simulink model "Driver_Fault_triggers"  (R2016a)
settings: Solver=VariableStepAuto  StartTime=0.0  StopTime=10.0  RelTol=1e-3
libraries: simulink x6
settings Model: Creator=ullek  LastModifiedBy=ullek

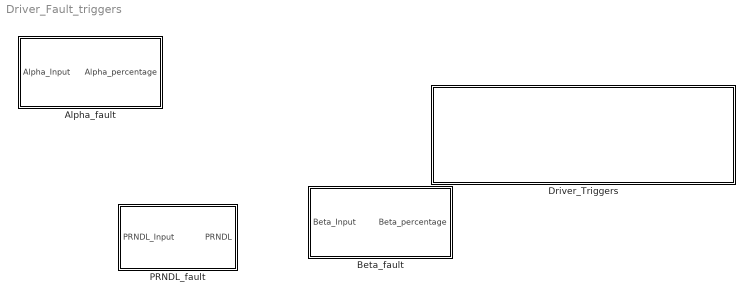
== system Driver_Fault_triggers ==
  Alpha_fault : Subsystem
  Beta_fault : Subsystem
  Driver_Triggers : Subsystem
  PRNDL_fault : Subsystem
  wires:
  ? -> Alpha_fault/1(Alpha_Input)  "Alpha_percentage"

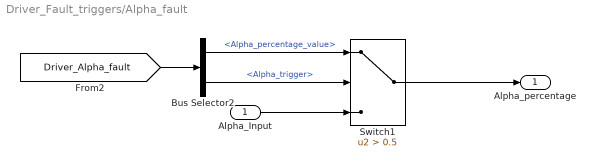
== system Driver_Fault_triggers/Alpha_fault ==
  Alpha_Input : Inport
  Bus Selector2 : BusSelector  OutputSignals=Alpha_percentage_value,Alpha_trigger
  Switch1 : Switch  Criteria=u2 > Threshold  Threshold=0.5
  Alpha_percentage : Outport
  wires:
  Alpha_Input/1 -> Switch1/3
  Switch1/1 -> Alpha_percentage/1
  Bus Selector2/2 -> Switch1/2  "<Alpha_trigger>"
  [Driver_Alpha_fault] -> Bus Selector2/1
  Bus Selector2/1 -> Switch1/1  "<Alpha_percentage_value>"

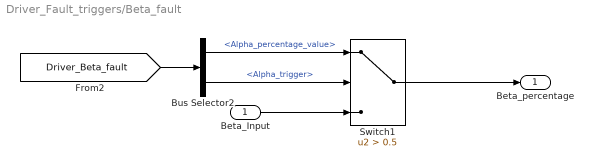
== system Driver_Fault_triggers/Beta_fault ==
  Beta_Input : Inport
  Bus Selector2 : BusSelector  OutputSignals=Alpha_percentage_value,Alpha_trigger
  Switch1 : Switch  Criteria=u2 > Threshold  Threshold=0.5
  Beta_percentage : Outport
  wires:
  Beta_Input/1 -> Switch1/3
  Switch1/1 -> Beta_percentage/1
  Bus Selector2/2 -> Switch1/2  "<Alpha_trigger>"
  [Driver_Beta_fault] -> Bus Selector2/1
  Bus Selector2/1 -> Switch1/1  "<Alpha_percentage_value>"

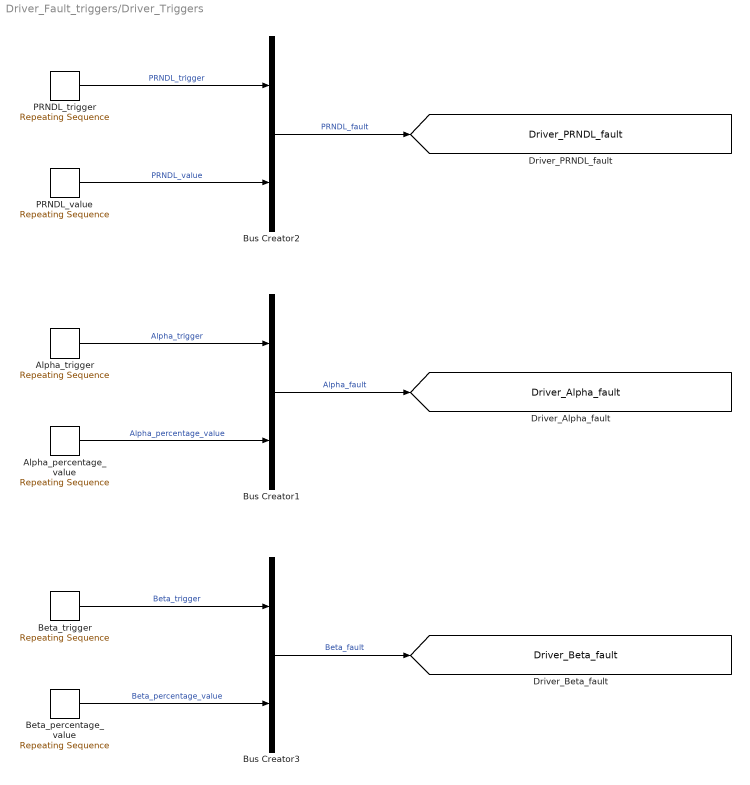
== system Driver_Fault_triggers/Driver_Triggers ==
  Alpha_percentage_value : simulink/Sources/Repeating Sequence  rep_seq_t=[0]  rep_seq_y=[0]
  Alpha_trigger : simulink/Sources/Repeating Sequence  rep_seq_t=[0]  rep_seq_y=[0]
  Beta_percentage_value : simulink/Sources/Repeating Sequence  rep_seq_t=[0]  rep_seq_y=[0]
  Beta_trigger : simulink/Sources/Repeating Sequence  rep_seq_t=[0]  rep_seq_y=[0]
  Bus Creator1 : BusCreator  Inputs=2
  Bus Creator2 : BusCreator  Inputs=2
  Bus Creator3 : BusCreator  Inputs=2
  PRNDL_trigger : simulink/Sources/Repeating Sequence  rep_seq_t=[0]  rep_seq_y=[0]
  PRNDL_value : simulink/Sources/Repeating Sequence  rep_seq_t=0  rep_seq_y=0
  tag scope: Driver_Alpha_fault=global, Driver_Beta_fault=global, Driver_PRNDL_fault=global
  wires:
  PRNDL_value/1 -> Bus Creator2/2  "PRNDL_value"
  Bus Creator2/1 -> [Driver_PRNDL_fault]  "PRNDL_fault"
  PRNDL_trigger/1 -> Bus Creator2/1  "PRNDL_trigger"
  Alpha_percentage_value/1 -> Bus Creator1/2  "Alpha_percentage_value"
  Bus Creator1/1 -> [Driver_Alpha_fault]  "Alpha_fault"
  Alpha_trigger/1 -> Bus Creator1/1  "Alpha_trigger"
  Beta_percentage_value/1 -> Bus Creator3/2  "Beta_percentage_value"
  Bus Creator3/1 -> [Driver_Beta_fault]  "Beta_fault"
  Beta_trigger/1 -> Bus Creator3/1  "Beta_trigger"

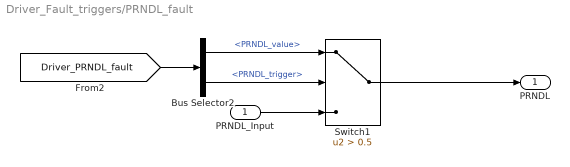
== system Driver_Fault_triggers/PRNDL_fault ==
  PRNDL_Input : Inport
  Bus Selector2 : BusSelector  OutputSignals=PRNDL_value,PRNDL_trigger
  Switch1 : Switch  Criteria=u2 > Threshold  Threshold=0.5
  PRNDL : Outport
  wires:
  PRNDL_Input/1 -> Switch1/3
  Switch1/1 -> PRNDL/1
  Bus Selector2/2 -> Switch1/2  "<PRNDL_trigger>"
  [Driver_PRNDL_fault] -> Bus Selector2/1
  Bus Selector2/1 -> Switch1/1  "<PRNDL_value>"
